simulink model "QuadrotorSimulink_expanded_breach"  (R2017a)
settings: Solver=ode45  StartTime=0.0  StopTime=tspan(end)  RelTol=1e-3  EnableMultiTasking=on
model workspace: external: MAT-File QuadrotorSimulink_expanded_params.mat (data not in the file)
undefined symbols (not defined in the file or in its folder): Quad
settings Model: Creator=test  LastModifiedBy=nikhil
settings DataIOCC: ExternalInput=[t__, u__]  SaveFormat=StructureWithTime  ReturnWorkspaceOutputs=on
settings OptimizationCC: ExpressionDepthLimit=2147483647  LifeSpan=inf
settings DebuggingCC: UnderspecifiedInitializationDetection=Classic  MergeDetectMultiDrivingBlocksExec=none  SolverPrmCheckMsg=warning  FcnCallInpInsideContextMsg=warning  StateNameClashWarn=warning  SFUnexpectedBacktrackingDiag=warning  SFNoUnconditionalDefaultTransitionDiag=warning  SFExecutionAtInitializationDiag=none
settings HardwareCC: ProdBitPerPointer=32  ProdBitPerSizeT=32  ProdBitPerPtrDiffT=32  ProdLargestAtomicFloat=None  ProdIntDivRoundTo=Undefined  ProdEndianess=Unspecified  ProdWordSize=32  ProdHWDeviceType=32-bit Generic
settings ModelReferenceCC: PropagateSignalLabelsOutOfModel=off
settings GRTTargetCC: TargetLangStandard=C89/C90 (ANSI)  CombineOutputUpdateFcns=off  GRTInterface=on
settings ConfigComp: CovMetricSettings=dw  CovHtmlReporting=on  CovSaveCumulativeToWorkspaceVar=on  CovSaveSingleToWorkspaceVar=on  CovExternalEMLEnable=off

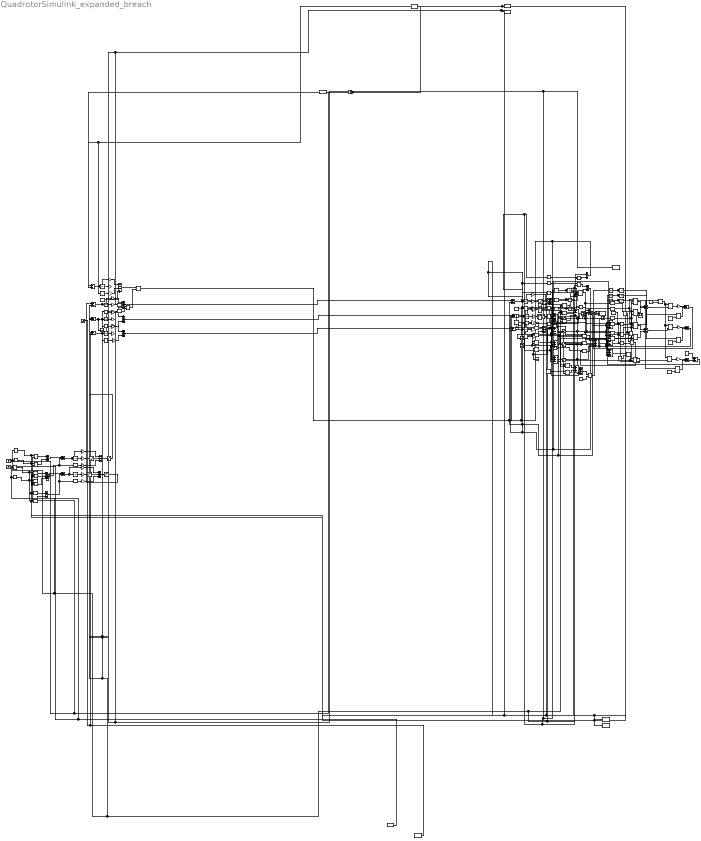
== system QuadrotorSimulink_expanded_breach ==
  note: YPID
  note: XPID
  note: PositionGFtoBF
  note: DesiredPositionGFtoBF
  note: TranslationalDynamics
  note: RotationalDynamics
  note: MotorSpeedCalculator
  note: AngularVelocitiesTransformation
  note: ZPID
  note: ThetaPID
  note: PsiPID
  note: PhiPID
  note: rPID
  note: qPID
  note: pPID
  note: TranslationalPositionPIDController
  note: QuadrotorSystem
  note: AttitudeAltitudePIDController
  note: AngularRatePIDController
  (Jx-Jy)/Jz : Constant  Value=(Quad.Jx - Quad.Jy)/Quad.Jz
  (Jy-Jz)/Jx : Constant  Value=(Quad.Jy - Quad.Jz)/Quad.Jx
  (Jz-Jx)/Jy : Constant  Value=(Quad.Jz - Quad.Jx)/Quad.Jy
  1/Jz : Constant  Value=1/Quad.Jz
  2*KT*l : Constant  Value=2*Quad.KT*Quad.l
  4*KT : Constant  Value=4*Quad.KT
  4*Kd : Constant  Value=4*Quad.Kd
  ActX : Integrator
  ActY : Integrator
  ActZ : Integrator
  Add : Sum  Inputs=+-+
  Add1 : Sum  Inputs=+++
  Add2 : Sum
  Derivative{,1..8} (9 alike) : Derivative
  Divide{,1..5} (6 alike) : Product  Inputs=*/
  Gain : Gain  Gain=-1
  Gain1 : Gain  Gain=-1
  Gain2 : Gain  Gain=-1
  Integrator{,1..8} (9 alike) : Integrator
  Jp : Constant  Value=Quad.Jp
  Jp/Jx : Constant  Value=Quad.Jp/Quad.Jx
  Jp/Jy : Constant  Value=Quad.Jp/Quad.Jy
  KT : Constant  Value=Quad.KT
  Kd : Gain  Gain=Quad.p_KD
  Kd1 : Gain  Gain=Quad.q_KD
  Kd2 : Gain  Gain=Quad.r_KD
  Kd3 : Gain  Gain=Quad.phi_KD
  Kd4 : Gain  Gain=Quad.psi_KD
  Kd5 : Gain  Gain=Quad.theta_KD
  Kd6 : Gain  Gain=Quad.Z_KD
  Kd7 : Constant  Value=Quad.Kd
  Kd8 : Gain  Gain=Quad.X_KD
  Kd9 : Gain  Gain=Quad.Y_KD
  Kdx/m : Constant  Value=Quad.Kdx/Quad.m
  Kdy/m : Constant  Value=Quad.Kdy/Quad.m
  Kdz/m : Constant  Value=Quad.Kdz/Quad.m
  Ki : Gain  Gain=Quad.p_KI
  Ki1 : Gain  Gain=Quad.q_KI
  Ki2 : Gain  Gain=Quad.r_KI
  Ki3 : Gain  Gain=Quad.phi_KI
  Ki4 : Gain  Gain=Quad.psi_KI
  Ki5 : Gain  Gain=Quad.theta_KI
  Ki6 : Gain  Gain=Quad.Z_KI
  Ki7 : Gain  Gain=Quad.X_KI
  Ki8 : Gain  Gain=Quad.Y_KI
  Kp : Gain  Gain=Quad.p_KP
  Kp1 : Gain  Gain=Quad.q_KP
  Kp2 : Gain  Gain=Quad.r_KP
  Kp3 : Gain  Gain=Quad.phi_KP
  Kp4 : Gain  Gain=Quad.psi_KP
  Kp5 : Gain  Gain=Quad.theta_KP
  Kp6 : Gain  Gain=Quad.Z_KP
  Kp7 : Gain  Gain=Quad.X_KP
  Kp8 : Gain  Gain=Quad.Y_KP
  OmegaBar : Sum  Inputs=+-+-
  Omegasqr1 : Sum  Inputs=+-+
  Omegasqr1cal : Sum  Inputs=++++
  Omegasqr2 : Sum  Inputs=+--
  Omegasqr2cal : Sum  Inputs=-+
  Omegasqr3 : Sum  Inputs=+++
  Omegasqr3cal : Sum  Inputs=-+
  Omegasqr4 : Sum  Inputs=++-
  Omegasqr4cal : Sum  Inputs=+-+-
  Phi : ToWorkspace  VariableName=Phi_out  SaveFormat=Structure  SampleTime=-1
  Phi1 : Integrator  ZeroCross=off
  Phidot : Integrator
  Product{,1,3,5..13} (12 alike) : Product  RndMeth=Zero
  Product2 : Product  Inputs=3  RndMeth=Zero
  Product4 : Product  Inputs=3  RndMeth=Zero
  ProductofElements{,1,3..4,6,11,13} (7 alike) : Product  Inputs=3
  ProductofElements{2,5,7..10,12,14..18} (12 alike) : Product
  Psi : ToWorkspace  VariableName=Psi_out  SaveFormat=Structure  SampleTime=-1
  Psi1 : Integrator  ZeroCross=off
  PsiError{,1..3} (4 alike) : Sum  Inputs=+-
  Psid : ToWorkspace  VariableName=Psi_desired  SaveFormat=Structure  SampleTime=-1
  Psidesired : Step  After=0  SampleTime=0
  Psidot : Integrator  ZeroCross=off
  Saturation{,3..5} (4 alike) : Saturate  UpperLimit=Quad.max_motor_speed^2  LowerLimit=Quad.min_motor_speed^2  ZeroCross=off
  Saturation1 : Saturate  UpperLimit=Quad.U2_max  LowerLimit=Quad.U2_min
  Saturation2 : Saturate  UpperLimit=Quad.U3_max  LowerLimit=Quad.U3_min
  Saturation6 : Saturate  UpperLimit=Quad.theta_max  LowerLimit=-Quad.theta_max
  Saturation7 : Saturate  UpperLimit=Quad.theta_max  LowerLimit=-Quad.theta_max
  Saturation8 : Saturate  UpperLimit=Quad.phi_max  LowerLimit=-Quad.phi_max
  Saturation9 : Saturate  UpperLimit=Quad.phi_max  LowerLimit=-Quad.phi_max
  Scope{,1..11} (12 alike) : Scope
  Sum{,1..5,15} (7 alike) : Sum  Inputs=+++
  Sum{8..10,12} (4 alike) : Sum
  Sum11 : Sum  Inputs=+-
  Sum13 : Sum  Inputs=+-
  Sum14 : Sum  Inputs=---
  Sum6 : Sum  Inputs=---+
  Sum7 : Sum  Inputs=+-
  Theta : ToWorkspace  VariableName=Theta_out  SaveFormat=Structure  SampleTime=-1
  Theta1 : Integrator  ZeroCross=off
  ThetaError : Sum  Inputs=+-
  Thetadot : Integrator  ZeroCross=off
  X : ToWorkspace  VariableName=X_out  SaveFormat=Structure  SampleTime=-1
  XError : Sum  Inputs=+-
  Xd : ToWorkspace  VariableName=X_desired  SaveFormat=Structure  SampleTime=-1
  Xdesired : Step  After=.25  SampleTime=0
  Xdot : Integrator
  Y : ToWorkspace  VariableName=Y_out  SaveFormat=Structure  SampleTime=-1
  YError : Sum  Inputs=+-
  Yd : ToWorkspace  VariableName=Y_desired  SaveFormat=Structure  SampleTime=-1
  Ydesired : Step  After=0  SampleTime=0
  Ydot : Integrator
  Z : ToWorkspace  VariableName=Z_out  SaveFormat=Structure  SampleTime=-1
  Zd : ToWorkspace  VariableName=Z_desired  SaveFormat=Structure  SampleTime=-1
  Zdesired : Step  After=.5  SampleTime=0
  Zdot : Integrator
  cosPhi : Trigonometry  Operator=cos
  cosPhi1 : Trigonometry  Operator=cos
  cosPsi : Trigonometry  Operator=cos
  cosTheta : Trigonometry  Operator=cos
  cosTheta1 : Trigonometry  Operator=cos
  ez : Sum  Inputs=+-
  g : Constant  Value=Quad.g
  l : Constant  Value=Quad.l
  l/Jx : Constant  Value=Quad.l/Quad.Jx
  l/Jy : Constant  Value=Quad.l/Quad.Jy
  m : Constant  Value=Quad.m
  mg : Constant  Value=Quad.m*Quad.g
  qError : Sum  Inputs=+-
  sin{,2..3,8,10} (5 alike) : Trigonometry
  sin{1,4..7,9} (6 alike) : Trigonometry  Operator=cos
  sinPhi : Trigonometry
  sinPsi : Trigonometry
  sinTheta : Trigonometry
  sum : Sum  Inputs=+-
  sum1 : Sum  Inputs=+-
  sum2 : Sum  Inputs=+-
  sum3 : Sum
  times{,1..6} (7 alike) : Product  Inputs=**
  ux : Sum
  uy : Sum  Inputs=+-
  wires:
  Add/1 -> Phidot/1
  Add2/1 -> Psidot/1
  sum3/1 -> Zdot/1
  sum1/1 -> Ydot/1
  sum/1 -> Xdot/1
  Add1/1 -> Thetadot/1
  Saturation1/1 -> Sum/2
  Ki/1 -> Saturation1/1
  Kd/1 -> Sum/3
  Integrator/1 -> Ki/1
  PsiError/1 -> Integrator/1, Kp/1
  Kp/1 -> Sum/1
  Derivative/1 -> Kd/1
  Sum3/1 -> PsiError/1
  Saturation2/1 -> Sum1/2
  Ki1/1 -> Saturation2/1
  Kd1/1 -> Sum1/3
  Integrator1/1 -> Ki1/1
  qError/1 -> Integrator1/1, Kp1/1, Scope/1
  Kp1/1 -> Sum1/1
  Derivative1/1 -> Kd1/1
  Sum5/1 -> qError/1
  Kd2/1 -> Sum2/3
  Integrator2/1 -> Ki2/1
  PsiError1/1 -> Integrator2/1, Kp2/1
  Kp2/1 -> Sum2/1
  Derivative2/1 -> Kd2/1
  Sum4/1 -> PsiError1/1
  Kd3/1 -> Sum3/3
  Integrator3/1 -> Ki3/1
  PsiError2/1 -> Integrator3/1, Kp3/1
  Kp3/1 -> Sum3/1
  Derivative3/1 -> Kd3/1
  Saturation9/1 -> PsiError2/1
  Kd4/1 -> Sum4/3
  Integrator4/1 -> Ki4/1
  PsiError3/1 -> Integrator4/1, Kp4/1
  Kp4/1 -> Sum4/1
  Derivative4/1 -> Kd4/1
  Psidesired/1 -> Psid/1, PsiError3/1  "Psi_desired"
  Kd5/1 -> Sum5/3
  Integrator5/1 -> Ki5/1
  ThetaError/1 -> Integrator5/1, Kp5/1, Scope1/1
  Kp5/1 -> Sum5/1
  Derivative5/1 -> Kd5/1
  Saturation7/1 -> ThetaError/1
  Kd6/1 -> Sum6/3
  mg/1 -> Sum6/4
  Sum6/1 -> Divide/1
  ez/1 -> Integrator6/1, Kp6/1
  Integrator6/1 -> Ki6/1
  Kp6/1 -> Sum6/1
  Derivative6/1 -> Kd6/1
  ActZ/1 -> ez/2, Derivative6/1, Z/1  "Z_out"
  Product/1 -> Divide/2
  cosTheta/1 -> Product/2
  cosPhi/1 -> Product/1
  Zdesired/1 -> ez/1, Zd/1  "Z_desired"
  Product4/1 -> Sum9/2
  Product3/1 -> Sum9/1
  sin6/1 -> Product4/3
  sin5/1 -> Product4/2
  sin3/1 -> Product3/2
  Product2/1 -> Sum8/2
  sin4/1 -> Product2/2
  sin2/1 -> Product2/1
  Product1/1 -> Sum8/1
  Thetadot/1 -> Product1/2, Product3/1, Theta1/1
  sin1/1 -> Product1/1
  Product5/1 -> Sum7/2
  Psidot/1 -> Product5/2, Product2/3, Product4/1, Psi1/1
  sin/1 -> Product5/1
  Phidot/1 -> Sum7/1, Phi1/1
  Omegasqr4/1 -> Saturation5/1
  Omegasqr3/1 -> Saturation3/1
  Omegasqr2/1 -> Saturation4/1
  Omegasqr1/1 -> Saturation/1
  Saturation4/1 -> OmegaBar/2, Omegasqr1cal/2, Omegasqr2cal/1, Omegasqr4cal/2, Scope6/1
  Saturation3/1 -> OmegaBar/3, Omegasqr1cal/3, Omegasqr3cal/2, Omegasqr4cal/3, Scope5/1
  Saturation5/1 -> OmegaBar/4, Omegasqr1cal/4, Omegasqr2cal/2, Omegasqr4cal/4, Scope4/1
  Saturation/1 -> OmegaBar/1, Omegasqr1cal/1, Omegasqr3cal/1, Omegasqr4cal/1, Scope7/1
  times2/1 -> times6/2
  times1/1 -> times5/2
  l/1 -> times5/1, times6/1
  Jp/1 -> times4/2
  Kd7/1 -> times3/2
  Omegasqr4cal/1 -> times3/1
  Omegasqr3cal/1 -> times2/2
  Omegasqr2cal/1 -> times1/2
  Omegasqr1cal/1 -> times/2
  KT/1 -> times/1, times1/1, times2/1
  OmegaBar/1 -> times4/1
  Divide1/1 -> Omegasqr2/2, Omegasqr4/2
  Divide3/1 -> Omegasqr1/3, Omegasqr2/3, Omegasqr3/3, Omegasqr4/3
  Divide2/1 -> Omegasqr1/2, Omegasqr3/2
  Divide4/1 -> Omegasqr1/1, Omegasqr2/1, Omegasqr3/1, Omegasqr4/1
  4*Kd/1 -> Divide3/2
  Sum2/1 -> Divide3/1, Scope2/1
  Sum1/1 -> Scope9/1, Divide2/1
  2*KT*l/1 -> Divide1/2, Divide2/2
  Sum/1 -> Scope8/1, Divide1/1
  4*KT/1 -> Divide4/2
  Divide/1 -> Scope10/1, Divide4/1
  ProductofElements6/1 -> Add2/1
  (Jx-Jy)/Jz/1 -> ProductofElements6/1
  1/Jz/1 -> ProductofElements7/1
  times3/1 -> Scope3/1, ProductofElements7/2
  ProductofElements7/1 -> Add2/2
  Sum7/1 -> PsiError/2, Derivative/1, ProductofElements3/2, ProductofElements4/2, ProductofElements6/2
  times6/1 -> ProductofElements5/2
  l/Jy/1 -> ProductofElements5/1
  Jp/Jy/1 -> ProductofElements4/1
  (Jz-Jx)/Jy/1 -> ProductofElements3/1
  ProductofElements5/1 -> Add1/3
  ProductofElements4/1 -> Add1/2
  ProductofElements3/1 -> Add1/1
  times4/1 -> ProductofElements1/3, ProductofElements4/3
  times5/1 -> ProductofElements2/2
  l/Jx/1 -> ProductofElements2/1
  Jp/Jx/1 -> ProductofElements1/1
  Sum9/1 -> PsiError1/2, Derivative2/1, ProductofElements/3, ProductofElements3/3
  Sum8/1 -> qError/2, Derivative1/1, ProductofElements/2, ProductofElements1/2, ProductofElements6/3
  (Jy-Jz)/Jx/1 -> ProductofElements/1
  ProductofElements2/1 -> Add/3
  ProductofElements1/1 -> Add/2
  ProductofElements/1 -> Add/1
  Gain2/1 -> sum2/1
  ProductofElements10/1 -> sum2/2
  sum2/1 -> sum3/2
  g/1 -> sum3/1
  ProductofElements18/1 -> Gain2/1
  Kdz/m/1 -> ProductofElements10/2
  Zdot/1 -> ProductofElements10/1, ActZ/1
  ProductofElements9/1 -> sum1/2
  Gain1/1 -> sum1/1
  Kdy/m/1 -> ProductofElements9/2
  Ydot/1 -> ProductofElements9/1, ActY/1
  ProductofElements8/1 -> sum/2
  Gain/1 -> sum/1
  Kdx/m/1 -> ProductofElements8/2
  Xdot/1 -> ProductofElements8/1, ActX/1
  ProductofElements17/1 -> Gain1/1
  ProductofElements16/1 -> Gain/1
  Divide5/1 -> ProductofElements16/1, ProductofElements17/1, ProductofElements18/1
  m/1 -> Divide5/2
  times/1 -> Divide5/1, Scope11/1
  ProductofElements15/1 -> ProductofElements18/2
  cosTheta1/1 -> ProductofElements15/2
  uy/1 -> ProductofElements17/2
  ProductofElements14/1 -> uy/2
  ProductofElements13/1 -> uy/1
  ux/1 -> ProductofElements16/2
  ProductofElements12/1 -> ux/2
  ProductofElements11/1 -> ux/1
  sinPsi/1 -> ProductofElements12/2, ProductofElements13/3
  sinPhi/1 -> ProductofElements12/1, ProductofElements14/1
  cosPhi1/1 -> ProductofElements11/1, ProductofElements13/1, ProductofElements15/1
  cosPsi/1 -> ProductofElements11/3, ProductofElements14/2
  sinTheta/1 -> ProductofElements11/2, ProductofElements13/2
  Theta1/1 -> sin4/1, sin6/1, sin/1, Theta/1, ThetaError/2, Derivative5/1, cosTheta/1, sinTheta/1, cosTheta1/1  "Theta_out"
  Phi1/1 -> sin3/1, sin5/1, sin1/1, sin2/1, PsiError2/2, Derivative3/1, cosPhi/1, Phi/1, sinPhi/1, cosPhi1/1  "Phi_out"
  Product9/1 -> Sum11/2
  Product8/1 -> Sum11/1
  Product7/1 -> Sum10/2
  Ydesired/1 -> Yd/1, Product7/2, Product8/2  "Y_desired"
  sin8/1 -> Product7/1, Product9/1
  Product6/1 -> Sum10/1
  Xdesired/1 -> Xd/1, Product6/2, Product9/2  "X_desired"
  sin7/1 -> Product6/1, Product8/1
  Product13/1 -> Sum13/2
  Product12/1 -> Sum13/1
  Product11/1 -> Sum12/2
  ActY/1 -> Product11/2, Product12/2, Y/1  "Y_out"
  sin10/1 -> Product11/1, Product13/1
  Product10/1 -> Sum12/1
  ActX/1 -> Product10/2, Product13/2, X/1  "X_out"
  sin9/1 -> Product10/1, Product12/1
  Psi1/1 -> PsiError3/2, Derivative4/1, sin9/1, sin10/1, sin7/1, sin8/1, Psi/1, sinPsi/1, cosPsi/1  "Psi_out"
  Saturation6/1 -> Sum14/2
  Ki7/1 -> Saturation6/1
  Kd8/1 -> Sum14/3
  Integrator7/1 -> Ki7/1
  XError/1 -> Integrator7/1, Kp7/1
  Sum14/1 -> Saturation7/1
  Kp7/1 -> Sum14/1
  Derivative7/1 -> Kd8/1
  Sum10/1 -> XError/1
  Sum12/1 -> XError/2, Derivative7/1
  Saturation8/1 -> Sum15/2
  Ki8/1 -> Saturation8/1
  Kd9/1 -> Sum15/3
  Integrator8/1 -> Ki8/1
  YError/1 -> Integrator8/1, Kp8/1
  Sum15/1 -> Saturation9/1
  Kp8/1 -> Sum15/1
  Derivative8/1 -> Kd9/1
  Sum11/1 -> YError/1
  Sum13/1 -> YError/2, Derivative8/1
